simulink model "DATA_Dictionarie_SMD_system"  (R2024b)
settings: Solver=VariableStepAuto  StartTime=0.0  StopTime=10.0  RelTol=1e-3
values from neighbouring files (symbols this model uses):
  b = 25.0    [Data11.sldd]    (also in Data22.sldd; data33.sldd)
  K = 3.0    [Data11.sldd]    (also in Data22.sldd; data33.sldd)
  M = 5.0    [Data11.sldd]    (also in Data22.sldd; data33.sldd)
settings Model: DataDictionary=datamix.sldd  Creator=chall  LastModifiedBy=chall

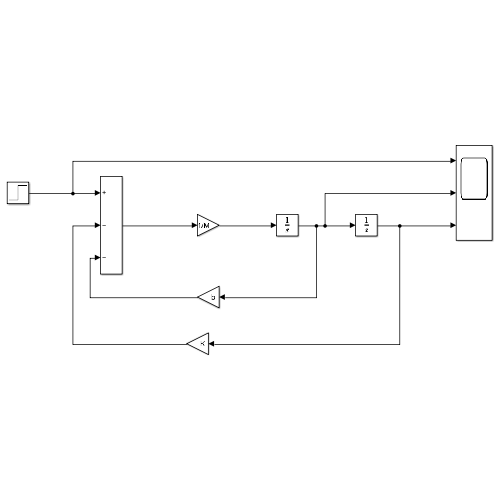
[thumbnail: Simulink's stored preview of the top-level diagram]
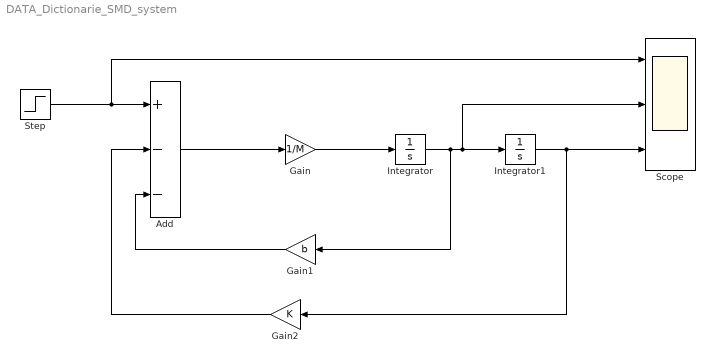
== system DATA_Dictionarie_SMD_system ==
  Add : Sum  Inputs=+--
  Gain : Gain  Gain=1/M
  Gain1 : Gain  Gain=b
  Gain2 : Gain  Gain=K
  Integrator : Integrator
  Integrator1 : Integrator
  Scope : Scope  NumInputPorts=3
  Step : Step  SampleTime=0
  wires:
  Integrator1/1 -> Gain2/1, Scope/3
  Step/1 -> Scope/1, Add/1
  Add/1 -> Gain/1
  Gain/1 -> Integrator/1
  Integrator/1 -> Gain1/1, Scope/2, Integrator1/1
  Gain1/1 -> Add/3
  Gain2/1 -> Add/2
